simulink model "MEMS_Gyro_Closed_SenseMode_yangchenglunwen"  (R2022b)
settings: Solver=FixedStepAuto  StartTime=0.0  StopTime=5  FixedStep=1/40000  MaxStep=1e-5  RelTol=1e-3
model workspace (MAT data in the model file):
  Ax = 5e-06
  Kamp = 210
  Kcv = 3.5
  Kyc = 114810
  Kyvf = 4.9943e-07
  Qy = 320
  Vr = 2
  Vref = 1
  a0 = 0
  a1 = -1.57079632679
  my = 6.7e-07
  wd = 24001.7678734
  wy = 24416.4581037
  wyx = 24001.7678734
libraries: slpidlib x10, dsparch4 x4
settings Model: Creator=Rio  LastModifiedBy=Rio

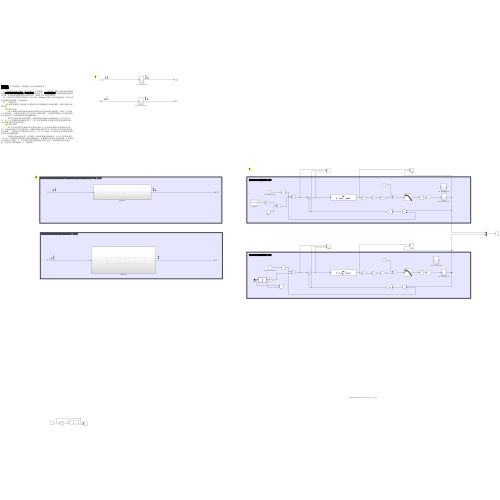
[thumbnail: Simulink's stored preview of the top-level diagram]
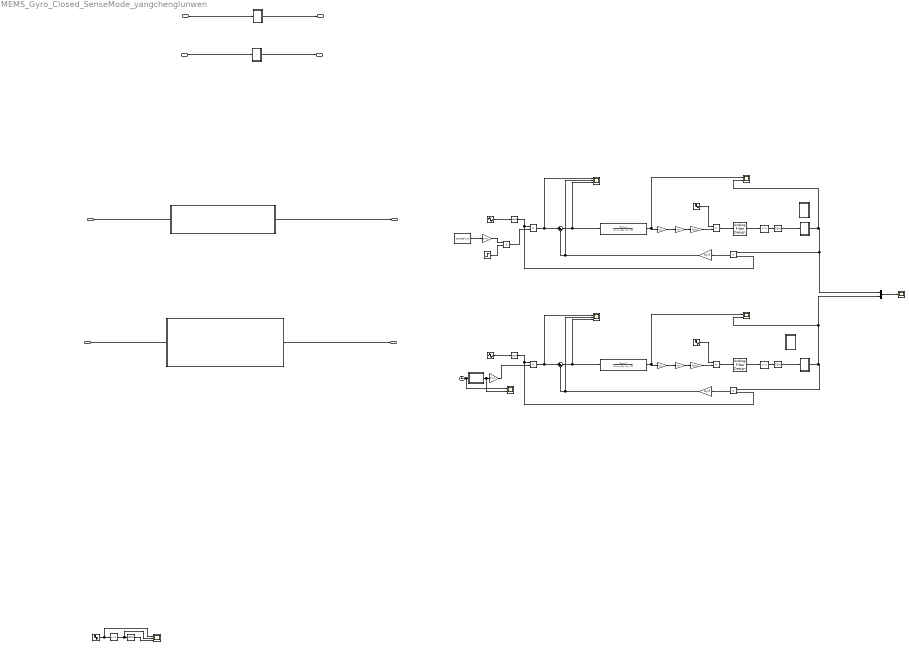
== system MEMS_Gyro_Closed_SenseMode_yangchenglunwen ==
  note: 1
  note: 模态匹配开环检测系统(时域)
  note: 仿真说明 ：参考杨成博士与詹超硕士论文闭环检测仿真
      | 仿真解释 ：
      | 1）闭环检测主要分为两个部分仿真，一个是频域，一个是时域。频域主要看闭环检测系统的 开环传递函数的伯德图、奈奎斯特图 分析稳定性。 闭环的伯德图 可以观察检测系统的带宽性能。时域就是直接观测给定输入信号，观测各个环节的响应情况。
      | 2）当前仿真均在模态匹配状态下进行仿真，即wy=wx,当输入恒定的角速度时，哥氏信号经检测模态相移90°，因此a=-90°。
      | 3）一共3类仿真：
      | 1 中对PI+串联校正器连续以及离散化后的传递函数进行观测伯德图，观察它幅频与相频特性；
      | 2 中有2个仿真：
      | 2.1 从频域传递函数角度观测闭环系统的开环传递函数的伯德图，加校正与不加校正环节的情形（目前仿出来和论文中是对得上的231122）。但是他的零极点与奈奎斯特图与论文相差较远（可能参数哪里有问题231122）。
      | 2.2 同时他的闭环系统伯德图，观测他的输出随输入的幅频特性与论文有很大出入，这一点与时域仿真是相相呼应的。（这与奈奎斯特图以及零极点图的特性是相符合的，因此参数可能还是存在问题）；
      | 3 中有2个仿真：
      | 3.1 首先从时域出发观测在稳定驱动位移信号与恒定角速度输入时系统输出的状态，这时候系统是可以闭环稳定的，检测位移基本被压到了0，加了校正环节后响应速度会有所减慢。（但是矫正环节输出的电压过大，与论文不太相符，可能还是存在参数或者那里结构有些问题231122）
      | 3.2 输入的角速度是有一定的频率，想观测其输出衰减情况，这与论文仿真结果有一定出入。检测反馈力随着输入角速度频率增大，在解调时可能会存在新的问题，这个需要在花些时间去理解一下。这与2.2中闭环的幅频特性是相对应的，说明是哪里还存在着问题，有时间还得仔细琢磨一下（231122）
  note: 观测开环检测输出随输入角速度频率变化，可反应带宽
  note: 3
  note: 模态匹配闭环检测系统的开环传递函数(校正与未校正环节对比)(频域)
  note: 模态匹配闭环检测系统的闭环观测（频域)
  note: 模态匹配开环检测系统(时域)
  note: 2
  Input2 : Inport
  In4 : Inport  Port=2
  Input1 : Inport  Port=3
  In1 : Inport  Port=4
  Analog Filter Design1 : dsparch4/Analog Filter Design  method=Butterworth  filttype=Lowpass  N=2  Wlo=2*pi*150  Whi=80  Rp=2  Rs=40
  Analog Filter Design3 : dsparch4/Analog Filter Design  method=Butterworth  filttype=Lowpass  N=2  Wlo=2*pi*150  Whi=80  Rp=2  Rs=40
  Clock2 : Clock
  Delay1 : Delay  SampleTime=1/1000
  Delay2 : Delay  SampleTime=1/40000
  Delay3 : Delay  SampleTime=1/40000
  Derivative : Derivative
  Derivative4 : Derivative
  Gain : Gain  Gain=2*my
  Gain1 : Gain  Gain=Kcv
  Gain10 : Gain  Gain=Kyc
  Gain11 : Gain  Gain=Kyvf
  Gain2 : Gain  Gain=Kamp
  Gain3 : Gain  Gain=Kyc
  Gain6 : Gain  Gain=Kyvf
  Gain7 : Gain  Gain=2*my
  Gain8 : Gain  Gain=Kcv
  Gain9 : Gain  Gain=Kamp
  MATLAB Function2 : MATLAB Function  TreatAsAtomicUnit=on
  Mux : Mux  Inputs=2
  Product{,1,8..11,13} (7 alike) : Product
  Scope : Scope  NumInputPorts=3
  Scope1 : Scope  NumInputPorts=3
  Scope10 : Scope  NumInputPorts=2
  Scope11 : Scope
  Scope2 : Scope  NumInputPorts=2
  Scope8 : Scope  NumInputPorts=3
  Scope9 : Scope  NumInputPorts=2
  Sine Wave : Sin  Frequency=2*pi*10  SampleTime=0
  Sine Wave1 : Sin  Frequency=wd  SampleTime=1/40000
  Sine Wave5 : Sin  Frequency=wd  SampleTime=1/40000
  Step : Step  SampleTime=1/40000
  Subsystem1 : Subsystem
  Subsystem2 : Subsystem
  Sum : Sum  Inputs=|+-
  Sum1 : Sum  Inputs=|+-
  Transfer Fcn : TransferFcn  Numerator=[1/my]  Denominator=[1 wyx/Qy wyx^2]
  Transfer Fcn2 : TransferFcn  Numerator=[1/my]  Denominator=[1 wyx/Qy wyx^2]
  Zero-Order Hold1 : ZeroOrderHold  SampleTime=1/1000
  Zero-Order Hold2 : ZeroOrderHold  SampleTime=1/40000
  Zero-Order Hold3 : ZeroOrderHold  SampleTime=1/40000
  离散：PI+串联校正器1 : Subsystem
  离散：PI+串联校正器2 : Subsystem
  离散：PI+串联校正器3 : Subsystem
  角速度输入 : Constant  Value=100/360*2*pi  SampleTime=1/40000
  连续：PI+串联校正器1 : Subsystem
  连续：PI+串联校正器2 : Subsystem
  连续：PI+串联校正器3 : Subsystem
  驱动模态速度位移输入 : Sin  Amplitude=Ax  Frequency=wd  SampleTime=1/40000
  驱动模态速度位移输入4 : Sin  Amplitude=Ax  Frequency=wd  SampleTime=1/40000
  Output2 : Outport
  Out4 : Outport  Port=2
  Output1 : Outport  Port=3
  Out1 : Outport  Port=4
  wires:
  Input2/1 -> 连续：PI+串联校正器1/1(u)
  连续：PI+串联校正器1/1(Output2) -> Output2/1
  驱动模态速度位移输入/1 -> Derivative/1
  角速度输入/1 -> Gain/1
  Derivative/1 -> Product9/2, Product/1
  Transfer Fcn/1 -> Gain3/1, Scope2/1
  Gain3/1 -> Gain1/1
  Gain1/1 -> Gain2/1
  Gain2/1 -> Product1/2
  Sine Wave1/1 -> Product1/1
  Product1/1 -> Analog Filter Design3/1
  In4/1 -> Subsystem1/1(In1)
  Subsystem1/1(Output2) -> Out4/1
  离散：PI+串联校正器2/1(Output2) -> Output1/1
  Input1/1 -> 离散：PI+串联校正器2/1(u)
  Delay1/1 -> Scope/2, Zero-Order Hold1/1
  Sine Wave/1 -> Scope/1, Delay1/1
  Zero-Order Hold1/1 -> Scope/3
  Subsystem2/1(Output2) -> Out1/1
  In1/1 -> Subsystem2/1(In1)
  Step/1 -> Product8/2
  Gain/1 -> Product8/1
  Product8/1 -> Product/2
  Product/1 -> Scope1/1, Sum/1
  Sum/1 -> Scope1/3, Transfer Fcn/1
  Product9/1 -> Gain6/1
  Gain6/1 -> Scope1/2, Sum/2
  Delay2/1 -> Zero-Order Hold2/1
  Analog Filter Design3/1 -> Delay2/1
  Zero-Order Hold2/1 -> 离散：PI+串联校正器1/1(u)
  离散：PI+串联校正器1/1(Output2) -> Scope2/2, Mux/1, Product9/1
  离散：PI+串联校正器3/1(Output2) -> Product13/1, Mux/2, Scope9/2
  Zero-Order Hold3/1 -> 离散：PI+串联校正器3/1(u)
  Analog Filter Design1/1 -> Delay3/1
  Delay3/1 -> Zero-Order Hold3/1
  Gain11/1 -> Sum1/2, Scope8/2
  Product13/1 -> Gain11/1
  Sum1/1 -> Transfer Fcn2/1, Scope8/3
  Product10/1 -> Sum1/1, Scope8/1
  Product11/1 -> Analog Filter Design1/1
  Sine Wave5/1 -> Product11/1
  Gain9/1 -> Product11/2
  Gain8/1 -> Gain9/1
  Gain10/1 -> Gain8/1
  Transfer Fcn2/1 -> Scope9/1, Gain10/1
  Derivative4/1 -> Product10/1, Product13/2
  驱动模态速度位移输入4/1 -> Derivative4/1
  MATLAB Function2/1(y) -> Gain7/1, Scope10/2
  Clock2/1 -> MATLAB Function2/1(u), Scope10/1
  Gain7/1 -> Product10/2
  Mux/1 -> Scope11/1

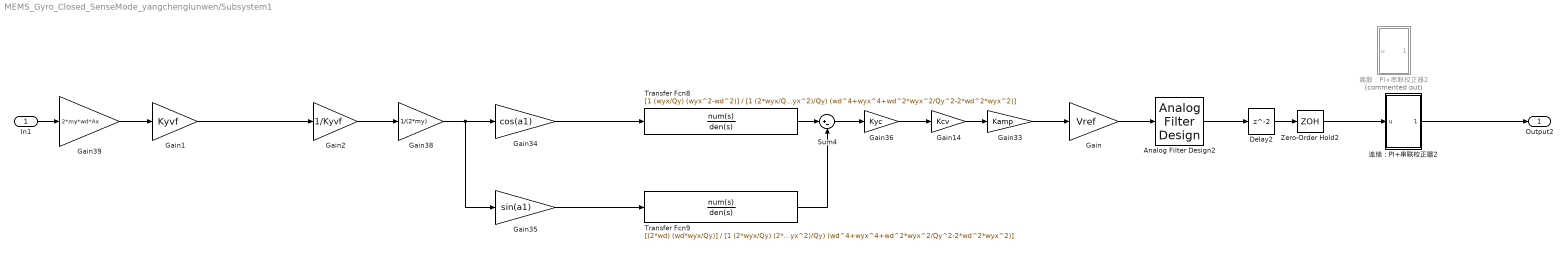
== system MEMS_Gyro_Closed_SenseMode_yangchenglunwen/Subsystem1 ==
  In1 : Inport
  Analog Filter Design2 : dsparch4/Analog Filter Design  method=Butterworth  filttype=Lowpass  N=2  Wlo=2*pi*150  Whi=80  Rp=2  Rs=40
  Delay2 : Delay  SampleTime=1/40000
  Gain : Gain  Gain=Vref
  Gain1 : Gain  Gain=Kyvf
  Gain14 : Gain  Gain=Kcv
  Gain2 : Gain  Gain=1/Kyvf
  Gain33 : Gain  Gain=Kamp
  Gain34 : Gain  Gain=cos(a1)
  Gain35 : Gain  Gain=sin(a1)
  Gain36 : Gain  Gain=Kyc
  Gain38 : Gain  Gain=1/(2*my)
  Gain39 : Gain  Gain=2*my*wd*Ax
  Sum4 : Sum  Inputs=|+-
  Transfer Fcn8 : TransferFcn  Numerator=[1 (wyx/Qy) (wyx^2-wd^2)]  Denominator=[1 (2*wyx/Qy) (2*wd^2+2*wyx^2+wyx^2/Qy^2) (2*wyx*(wd^2+wyx^2)/Qy) (wd^4+wyx^4+wd^2*wyx^2/Qy^2-2*wd^2*wyx^2)]
  Transfer Fcn9 : TransferFcn  Numerator=[(2*wd) (wd*wyx/Qy)]  Denominator=[1 (2*wyx/Qy) (2*wd^2+2*wyx^2+wyx^2/Qy^2) (2*wyx*(wd^2+wyx^2)/Qy) (wd^4+wyx^4+wd^2*wyx^2/Qy^2-2*wd^2*wyx^2)]
  Zero-Order Hold2 : ZeroOrderHold  SampleTime=1/40000
  离散：PI+串联校正器2 : Subsystem  Commented=on
  连续：PI+串联校正器2 : Subsystem
  Output2 : Outport
  wires:
  Analog Filter Design2/1 -> Delay2/1
  Delay2/1 -> Zero-Order Hold2/1
  Sum4/1 -> Gain36/1
  Gain38/1 -> Gain34/1, Gain35/1
  Gain34/1 -> Transfer Fcn8/1
  Transfer Fcn8/1 -> Sum4/1
  Transfer Fcn9/1 -> Sum4/2
  Gain14/1 -> Gain33/1
  Gain35/1 -> Transfer Fcn9/1
  Gain36/1 -> Gain14/1
  In1/1 -> Gain39/1
  Gain33/1 -> Gain/1
  Gain/1 -> Analog Filter Design2/1
  Gain39/1 -> Gain1/1
  Gain2/1 -> Gain38/1
  Zero-Order Hold2/1 -> 连续：PI+串联校正器2/1(u)
  连续：PI+串联校正器2/1(Output2) -> Output2/1
  Gain1/1 -> Gain2/1

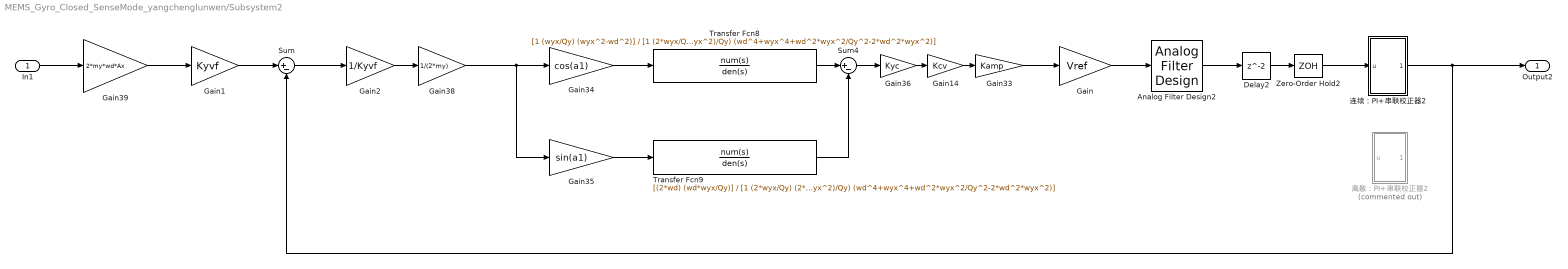
== system MEMS_Gyro_Closed_SenseMode_yangchenglunwen/Subsystem2 ==
  In1 : Inport
  Analog Filter Design2 : dsparch4/Analog Filter Design  method=Butterworth  filttype=Lowpass  N=2  Wlo=2*pi*150  Whi=80  Rp=2  Rs=40
  Delay2 : Delay  SampleTime=1/1000
  Gain : Gain  Gain=Vref
  Gain1 : Gain  Gain=Kyvf
  Gain14 : Gain  Gain=Kcv
  Gain2 : Gain  Gain=1/Kyvf
  Gain33 : Gain  Gain=Kamp
  Gain34 : Gain  Gain=cos(a1)
  Gain35 : Gain  Gain=sin(a1)
  Gain36 : Gain  Gain=Kyc
  Gain38 : Gain  Gain=1/(2*my)
  Gain39 : Gain  Gain=2*my*wd*Ax
  Sum : Sum  Inputs=|+-
  Sum4 : Sum  Inputs=|+-
  Transfer Fcn8 : TransferFcn  Numerator=[1 (wyx/Qy) (wyx^2-wd^2)]  Denominator=[1 (2*wyx/Qy) (2*wd^2+2*wyx^2+wyx^2/Qy^2) (2*wyx*(wd^2+wyx^2)/Qy) (wd^4+wyx^4+wd^2*wyx^2/Qy^2-2*wd^2*wyx^2)]
  Transfer Fcn9 : TransferFcn  Numerator=[(2*wd) (wd*wyx/Qy)]  Denominator=[1 (2*wyx/Qy) (2*wd^2+2*wyx^2+wyx^2/Qy^2) (2*wyx*(wd^2+wyx^2)/Qy) (wd^4+wyx^4+wd^2*wyx^2/Qy^2-2*wd^2*wyx^2)]
  Zero-Order Hold2 : ZeroOrderHold  SampleTime=1/1000
  离散：PI+串联校正器2 : Subsystem  Commented=on
  连续：PI+串联校正器2 : Subsystem
  Output2 : Outport
  wires:
  Analog Filter Design2/1 -> Delay2/1
  Gain/1 -> Analog Filter Design2/1
  Gain33/1 -> Gain/1
  In1/1 -> Gain39/1
  Sum4/1 -> Gain36/1
  Gain36/1 -> Gain14/1
  Gain34/1 -> Transfer Fcn8/1
  Gain35/1 -> Transfer Fcn9/1
  Transfer Fcn9/1 -> Sum4/2
  Transfer Fcn8/1 -> Sum4/1
  Delay2/1 -> Zero-Order Hold2/1
  连续：PI+串联校正器2/1(Output2) -> Sum/2, Output2/1
  Gain14/1 -> Gain33/1
  Gain38/1 -> Gain35/1, Gain34/1
  Zero-Order Hold2/1 -> 连续：PI+串联校正器2/1(u)
  Gain39/1 -> Gain1/1
  Gain1/1 -> Sum/1
  Gain2/1 -> Gain38/1
  Sum/1 -> Gain2/1

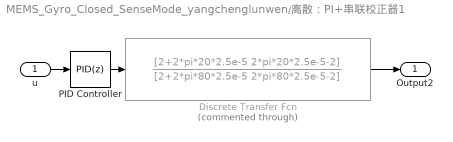
== system MEMS_Gyro_Closed_SenseMode_yangchenglunwen/离散：PI+串联校正器1 ==
  u : Inport
  Discrete Transfer Fcn : DiscreteTransferFcn  Commented=through  Numerator=[2+2*pi*20*2.5e-5 2*pi*20*2.5e-5-2]  Denominator=[2+2*pi*80*2.5e-5 2*pi*80*2.5e-5-2]  SampleTime=1/40000
  PID Controller : slpidlib/PID Controller  Controller=PID  Form=Parallel  TimeDomain=Discrete-time  UseExternalTs=off  SampleTime=1/40000  IntegratorMethod=Forward Euler  FilterMethod=Forward Euler  ControllerParametersSource=internal  P=0.1  I=2*pi*20  UseKiTs=off  D=0  N=100  UseFilter=on  TunerSelectOption=Transfer Function Based (PID Tuner App)  InitialConditionSource=internal  InitialConditionForIntegrator=0  InitialConditionForFilter=0  DifferentiatorICPrevScaledInput=0  ExternalReset=none  TrackingMode=off  Kt=1  LimitOutput=off  SatLimitsSource=internal  UpperSaturationLimit=inf  LowerSaturationLimit=-inf  LinearizeAsGain=on  AntiWindupMode=none  Kb=1  LimitIntegrator=off  UpperIntegratorSaturationLimit=inf  LowerIntegratorSaturationLimit=-inf  POutMin=[]  POutMax=[]  IOutMin=[]  IOutMax=[]  DOutMin=[]  DOutMax=[]  NOutMin=[]  NOutMax=[]  SumOutMin=[]  SumOutMax=[]  SaturationOutMin=[]  SaturationOutMax=[]  PParamMin=[]  PParamMax=[]  IParamMin=[]  IParamMax=[]  DParamMin=[]  DParamMax=[]  NParamMin=[]  NParamMax=[]  KbParamMin=[]  KbParamMax=[]  KtParamMin=[]  KtParamMax=[]  KbOutMin=[]  KbOutMax=[]  KtOutMin=[]  KtOutMax=[]  IntegratorOutMin=[]  IntegratorOutMax=[]  FilterOutMin=[]  FilterOutMax=[]  SumI1OutMin=[]  SumI1OutMax=[]  SumI2OutMin=[]  SumI2OutMax=[]  SumI3OutMin=[]  SumI3OutMax=[]  SumI4OutMin=[]  SumI4OutMax=[]  SumDOutMin=[]  SumDOutMax=[]  DifferentiatorOutMin=[]  DifferentiatorOutMax=[]  FilterDiffOutCoefMin=[]  FilterDiffOutCoefMax=[]  ReciprocalOutMin=[]  ReciprocalOutMax=[]  SumDenOutMin=[]  SumDenOutMax=[]  SumNumOutMin=[]  SumNumOutMax=[]  DivideOutMin=[]  DivideOutMax=[]  UdiffTsProdOutMin=[]  UdiffTsProdOutMax=[]  NTsProdOutMin=[]  NTsProdOutMax=[]  UintegralTsProdOutMin=[]  UintegralTsProdOutMax=[]  UngainTsProdOutMin=[]  UngainTsProdOutMax=[]  ClampingZeroOutDataTypeStr=Inherit: Inherit via back propagation  ClampingZeroOutMin=[]  ClampingZeroOutMax=[]  FilterDenConstantOutDataTypeStr=Inherit: Inherit via back propagation  FilterDenConstantOutMin=[]  FilterDenConstantOutMax=[]  PCopyOutDataTypeStr=Inherit: Inherit via back propagation  PCopyOutMin=[]  PCopyOutMax=[]  NCopyOutDataTypeStr=Inherit: Inherit via back propagation  NCopyOutMin=[]  NCopyOutMax=[]  IntegratorContinuousStateAttributes=''  IntegratorStateMustResolveToSignalObject=off  IntegratorRTWStateStorageClass=Auto  FilterContinuousStateAttributes=''  FilterStateMustResolveToSignalObject=off  FilterRTWStateStorageClass=Auto  ParallelPVariant=InternalParameters  IdealPVariant=Disabled  IVariant=InternalParameters  DVariant=InternalParameters  IntegratorVariant=Discrete  SatVariant=Disabled  AWVariant=Passthrough  PCopyVariant=Disabled  TRVariant=Disabled  FdbkBlocksVariant=Forward  IdealPFdbkVariant=Disabled  SatFdbkVariant=Disabled  DerivativeFilterVariant=ForwardEulerFilter  NVariant=InternalParameters  NCopyVariant=Disabled  FilterICVariant=InternalICsFilter  IntegratorICVariant=InternalICs  ExternalResetVariant=Disabled  TRSumVariant=Passthrough  SumFdbkVariant=Disabled  SumVariant=Sum_PID  TsampFilterVariant=InternalTs  TsampNgainVariant=Passthrough  TsampIntegralVariant=Passthrough  ExternalSaturationOutDataTypeStr=Inherit: Same as second input
  Output2 : Outport
  wires:
  Discrete Transfer Fcn/1 -> Output2/1
  PID Controller/1 -> Discrete Transfer Fcn/1
  u/1 -> PID Controller/1

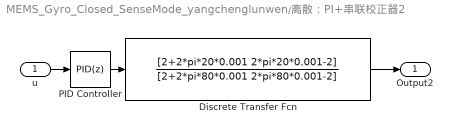
== system MEMS_Gyro_Closed_SenseMode_yangchenglunwen/离散：PI+串联校正器2 ==
  u : Inport
  Discrete Transfer Fcn : DiscreteTransferFcn  Numerator=[2+2*pi*20*0.001 2*pi*20*0.001-2]  Denominator=[2+2*pi*80*0.001 2*pi*80*0.001-2]
  PID Controller : slpidlib/PID Controller  Controller=PID  Form=Parallel  TimeDomain=Discrete-time  UseExternalTs=off  SampleTime=1/1000  IntegratorMethod=Forward Euler  FilterMethod=Forward Euler  ControllerParametersSource=internal  P=0.9  I=2*pi*18  UseKiTs=off  D=0  N=100  UseFilter=on  TunerSelectOption=Transfer Function Based (PID Tuner App)  InitialConditionSource=internal  InitialConditionForIntegrator=0  InitialConditionForFilter=0  DifferentiatorICPrevScaledInput=0  ExternalReset=none  TrackingMode=off  Kt=1  LimitOutput=off  SatLimitsSource=internal  UpperSaturationLimit=inf  LowerSaturationLimit=-inf  LinearizeAsGain=on  AntiWindupMode=none  Kb=1  LimitIntegrator=off  UpperIntegratorSaturationLimit=inf  LowerIntegratorSaturationLimit=-inf  POutMin=[]  POutMax=[]  IOutMin=[]  IOutMax=[]  DOutMin=[]  DOutMax=[]  NOutMin=[]  NOutMax=[]  SumOutMin=[]  SumOutMax=[]  SaturationOutMin=[]  SaturationOutMax=[]  PParamMin=[]  PParamMax=[]  IParamMin=[]  IParamMax=[]  DParamMin=[]  DParamMax=[]  NParamMin=[]  NParamMax=[]  KbParamMin=[]  KbParamMax=[]  KtParamMin=[]  KtParamMax=[]  KbOutMin=[]  KbOutMax=[]  KtOutMin=[]  KtOutMax=[]  IntegratorOutMin=[]  IntegratorOutMax=[]  FilterOutMin=[]  FilterOutMax=[]  SumI1OutMin=[]  SumI1OutMax=[]  SumI2OutMin=[]  SumI2OutMax=[]  SumI3OutMin=[]  SumI3OutMax=[]  SumI4OutMin=[]  SumI4OutMax=[]  SumDOutMin=[]  SumDOutMax=[]  DifferentiatorOutMin=[]  DifferentiatorOutMax=[]  FilterDiffOutCoefMin=[]  FilterDiffOutCoefMax=[]  ReciprocalOutMin=[]  ReciprocalOutMax=[]  SumDenOutMin=[]  SumDenOutMax=[]  SumNumOutMin=[]  SumNumOutMax=[]  DivideOutMin=[]  DivideOutMax=[]  UdiffTsProdOutMin=[]  UdiffTsProdOutMax=[]  NTsProdOutMin=[]  NTsProdOutMax=[]  UintegralTsProdOutMin=[]  UintegralTsProdOutMax=[]  UngainTsProdOutMin=[]  UngainTsProdOutMax=[]  ClampingZeroOutDataTypeStr=Inherit: Inherit via back propagation  ClampingZeroOutMin=[]  ClampingZeroOutMax=[]  FilterDenConstantOutDataTypeStr=Inherit: Inherit via back propagation  FilterDenConstantOutMin=[]  FilterDenConstantOutMax=[]  PCopyOutDataTypeStr=Inherit: Inherit via back propagation  PCopyOutMin=[]  PCopyOutMax=[]  NCopyOutDataTypeStr=Inherit: Inherit via back propagation  NCopyOutMin=[]  NCopyOutMax=[]  IntegratorContinuousStateAttributes=''  IntegratorStateMustResolveToSignalObject=off  IntegratorRTWStateStorageClass=Auto  FilterContinuousStateAttributes=''  FilterStateMustResolveToSignalObject=off  FilterRTWStateStorageClass=Auto  ParallelPVariant=InternalParameters  IdealPVariant=Disabled  IVariant=InternalParameters  DVariant=InternalParameters  IntegratorVariant=Discrete  SatVariant=Disabled  AWVariant=Passthrough  PCopyVariant=Disabled  TRVariant=Disabled  FdbkBlocksVariant=Forward  IdealPFdbkVariant=Disabled  SatFdbkVariant=Disabled  DerivativeFilterVariant=ForwardEulerFilter  NVariant=InternalParameters  NCopyVariant=Disabled  FilterICVariant=InternalICsFilter  IntegratorICVariant=InternalICs  ExternalResetVariant=Disabled  TRSumVariant=Passthrough  SumFdbkVariant=Disabled  SumVariant=Sum_PID  TsampFilterVariant=InternalTs  TsampNgainVariant=Passthrough  TsampIntegralVariant=Passthrough  ExternalSaturationOutDataTypeStr=Inherit: Same as second input
  Output2 : Outport
  wires:
  u/1 -> PID Controller/1
  PID Controller/1 -> Discrete Transfer Fcn/1
  Discrete Transfer Fcn/1 -> Output2/1

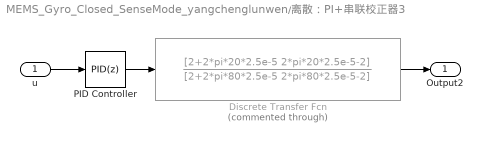
== system MEMS_Gyro_Closed_SenseMode_yangchenglunwen/离散：PI+串联校正器3 ==
  u : Inport
  Discrete Transfer Fcn : DiscreteTransferFcn  Commented=through  Numerator=[2+2*pi*20*2.5e-5 2*pi*20*2.5e-5-2]  Denominator=[2+2*pi*80*2.5e-5 2*pi*80*2.5e-5-2]  SampleTime=1/40000
  PID Controller : slpidlib/PID Controller  Controller=PID  Form=Parallel  TimeDomain=Discrete-time  UseExternalTs=off  SampleTime=1/40000  IntegratorMethod=Forward Euler  FilterMethod=Forward Euler  ControllerParametersSource=internal  P=0.1  I=2*pi*20  UseKiTs=off  D=0  N=100  UseFilter=on  TunerSelectOption=Transfer Function Based (PID Tuner App)  InitialConditionSource=internal  InitialConditionForIntegrator=0  InitialConditionForFilter=0  DifferentiatorICPrevScaledInput=0  ExternalReset=none  TrackingMode=off  Kt=1  LimitOutput=off  SatLimitsSource=internal  UpperSaturationLimit=inf  LowerSaturationLimit=-inf  LinearizeAsGain=on  AntiWindupMode=none  Kb=1  LimitIntegrator=off  UpperIntegratorSaturationLimit=inf  LowerIntegratorSaturationLimit=-inf  POutMin=[]  POutMax=[]  IOutMin=[]  IOutMax=[]  DOutMin=[]  DOutMax=[]  NOutMin=[]  NOutMax=[]  SumOutMin=[]  SumOutMax=[]  SaturationOutMin=[]  SaturationOutMax=[]  PParamMin=[]  PParamMax=[]  IParamMin=[]  IParamMax=[]  DParamMin=[]  DParamMax=[]  NParamMin=[]  NParamMax=[]  KbParamMin=[]  KbParamMax=[]  KtParamMin=[]  KtParamMax=[]  KbOutMin=[]  KbOutMax=[]  KtOutMin=[]  KtOutMax=[]  IntegratorOutMin=[]  IntegratorOutMax=[]  FilterOutMin=[]  FilterOutMax=[]  SumI1OutMin=[]  SumI1OutMax=[]  SumI2OutMin=[]  SumI2OutMax=[]  SumI3OutMin=[]  SumI3OutMax=[]  SumI4OutMin=[]  SumI4OutMax=[]  SumDOutMin=[]  SumDOutMax=[]  DifferentiatorOutMin=[]  DifferentiatorOutMax=[]  FilterDiffOutCoefMin=[]  FilterDiffOutCoefMax=[]  ReciprocalOutMin=[]  ReciprocalOutMax=[]  SumDenOutMin=[]  SumDenOutMax=[]  SumNumOutMin=[]  SumNumOutMax=[]  DivideOutMin=[]  DivideOutMax=[]  UdiffTsProdOutMin=[]  UdiffTsProdOutMax=[]  NTsProdOutMin=[]  NTsProdOutMax=[]  UintegralTsProdOutMin=[]  UintegralTsProdOutMax=[]  UngainTsProdOutMin=[]  UngainTsProdOutMax=[]  ClampingZeroOutDataTypeStr=Inherit: Inherit via back propagation  ClampingZeroOutMin=[]  ClampingZeroOutMax=[]  FilterDenConstantOutDataTypeStr=Inherit: Inherit via back propagation  FilterDenConstantOutMin=[]  FilterDenConstantOutMax=[]  PCopyOutDataTypeStr=Inherit: Inherit via back propagation  PCopyOutMin=[]  PCopyOutMax=[]  NCopyOutDataTypeStr=Inherit: Inherit via back propagation  NCopyOutMin=[]  NCopyOutMax=[]  IntegratorContinuousStateAttributes=''  IntegratorStateMustResolveToSignalObject=off  IntegratorRTWStateStorageClass=Auto  FilterContinuousStateAttributes=''  FilterStateMustResolveToSignalObject=off  FilterRTWStateStorageClass=Auto  ParallelPVariant=InternalParameters  IdealPVariant=Disabled  IVariant=InternalParameters  DVariant=InternalParameters  IntegratorVariant=Discrete  SatVariant=Disabled  AWVariant=Passthrough  PCopyVariant=Disabled  TRVariant=Disabled  FdbkBlocksVariant=Forward  IdealPFdbkVariant=Disabled  SatFdbkVariant=Disabled  DerivativeFilterVariant=ForwardEulerFilter  NVariant=InternalParameters  NCopyVariant=Disabled  FilterICVariant=InternalICsFilter  IntegratorICVariant=InternalICs  ExternalResetVariant=Disabled  TRSumVariant=Passthrough  SumFdbkVariant=Disabled  SumVariant=Sum_PID  TsampFilterVariant=InternalTs  TsampNgainVariant=Passthrough  TsampIntegralVariant=Passthrough  ExternalSaturationOutDataTypeStr=Inherit: Same as second input
  Output2 : Outport
  wires:
  u/1 -> PID Controller/1
  PID Controller/1 -> Discrete Transfer Fcn/1
  Discrete Transfer Fcn/1 -> Output2/1

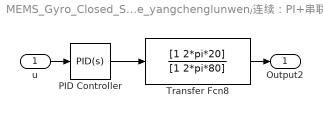
== system MEMS_Gyro_Closed_SenseMode_yangchenglunwen/连续：PI+串联校正器1 ==
  u : Inport
  PID Controller : slpidlib/PID Controller  Controller=PID  Form=Parallel  TimeDomain=Continuous-time  UseExternalTs=off  SampleTime=-1  IntegratorMethod=Forward Euler  FilterMethod=Forward Euler  ControllerParametersSource=internal  P=0.9  I=2*pi*18  UseKiTs=off  D=0  N=100  UseFilter=on  TunerSelectOption=Transfer Function Based (PID Tuner App)  InitialConditionSource=internal  InitialConditionForIntegrator=0  InitialConditionForFilter=0  DifferentiatorICPrevScaledInput=0  ExternalReset=none  TrackingMode=off  Kt=1  LimitOutput=off  SatLimitsSource=internal  UpperSaturationLimit=inf  LowerSaturationLimit=-inf  LinearizeAsGain=on  AntiWindupMode=none  Kb=1  LimitIntegrator=off  UpperIntegratorSaturationLimit=inf  LowerIntegratorSaturationLimit=-inf  POutMin=[]  POutMax=[]  IOutMin=[]  IOutMax=[]  DOutMin=[]  DOutMax=[]  NOutMin=[]  NOutMax=[]  SumOutMin=[]  SumOutMax=[]  SaturationOutMin=[]  SaturationOutMax=[]  PParamMin=[]  PParamMax=[]  IParamMin=[]  IParamMax=[]  DParamMin=[]  DParamMax=[]  NParamMin=[]  NParamMax=[]  KbParamMin=[]  KbParamMax=[]  KtParamMin=[]  KtParamMax=[]  KbOutMin=[]  KbOutMax=[]  KtOutMin=[]  KtOutMax=[]  IntegratorOutMin=[]  IntegratorOutMax=[]  FilterOutMin=[]  FilterOutMax=[]  SumI1OutMin=[]  SumI1OutMax=[]  SumI2OutMin=[]  SumI2OutMax=[]  SumI3OutMin=[]  SumI3OutMax=[]  SumI4OutMin=[]  SumI4OutMax=[]  SumDOutMin=[]  SumDOutMax=[]  DifferentiatorOutMin=[]  DifferentiatorOutMax=[]  FilterDiffOutCoefMin=[]  FilterDiffOutCoefMax=[]  ReciprocalOutMin=[]  ReciprocalOutMax=[]  SumDenOutMin=[]  SumDenOutMax=[]  SumNumOutMin=[]  SumNumOutMax=[]  DivideOutMin=[]  DivideOutMax=[]  UdiffTsProdOutMin=[]  UdiffTsProdOutMax=[]  NTsProdOutMin=[]  NTsProdOutMax=[]  UintegralTsProdOutMin=[]  UintegralTsProdOutMax=[]  UngainTsProdOutMin=[]  UngainTsProdOutMax=[]  ClampingZeroOutDataTypeStr=Inherit: Inherit via back propagation  ClampingZeroOutMin=[]  ClampingZeroOutMax=[]  FilterDenConstantOutDataTypeStr=Inherit: Inherit via back propagation  FilterDenConstantOutMin=[]  FilterDenConstantOutMax=[]  PCopyOutDataTypeStr=Inherit: Inherit via back propagation  PCopyOutMin=[]  PCopyOutMax=[]  NCopyOutDataTypeStr=Inherit: Inherit via back propagation  NCopyOutMin=[]  NCopyOutMax=[]  IntegratorContinuousStateAttributes=''  IntegratorStateMustResolveToSignalObject=off  IntegratorRTWStateStorageClass=Auto  FilterContinuousStateAttributes=''  FilterStateMustResolveToSignalObject=off  FilterRTWStateStorageClass=Auto  ParallelPVariant=InternalParameters  IdealPVariant=Disabled  IVariant=InternalParameters  DVariant=InternalParameters  IntegratorVariant=Continuous  SatVariant=Disabled  AWVariant=Passthrough  PCopyVariant=Disabled  TRVariant=Disabled  FdbkBlocksVariant=Forward  IdealPFdbkVariant=Disabled  SatFdbkVariant=Disabled  DerivativeFilterVariant=ContFilter  NVariant=InternalParameters  NCopyVariant=Disabled  FilterICVariant=InternalICsFilter  IntegratorICVariant=InternalICs  ExternalResetVariant=Disabled  TRSumVariant=Passthrough  SumFdbkVariant=Disabled  SumVariant=Sum_PID  TsampFilterVariant=InternalTs  TsampNgainVariant=Passthrough  TsampIntegralVariant=Passthrough  ExternalSaturationOutDataTypeStr=Inherit: Same as second input
  Transfer Fcn8 : TransferFcn  Numerator=[1 2*pi*20]  Denominator=[1 2*pi*80]
  Output2 : Outport
  wires:
  Transfer Fcn8/1 -> Output2/1
  PID Controller/1 -> Transfer Fcn8/1
  u/1 -> PID Controller/1

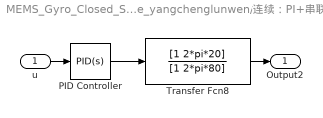
== system MEMS_Gyro_Closed_SenseMode_yangchenglunwen/连续：PI+串联校正器2 ==
  u : Inport
  PID Controller : slpidlib/PID Controller  Controller=PID  Form=Parallel  TimeDomain=Continuous-time  UseExternalTs=off  SampleTime=-1  IntegratorMethod=Forward Euler  FilterMethod=Forward Euler  ControllerParametersSource=internal  P=0.9  I=2*pi*18  UseKiTs=off  D=0  N=100  UseFilter=on  TunerSelectOption=Transfer Function Based (PID Tuner App)  InitialConditionSource=internal  InitialConditionForIntegrator=0  InitialConditionForFilter=0  DifferentiatorICPrevScaledInput=0  ExternalReset=none  TrackingMode=off  Kt=1  LimitOutput=off  SatLimitsSource=internal  UpperSaturationLimit=inf  LowerSaturationLimit=-inf  LinearizeAsGain=on  AntiWindupMode=none  Kb=1  LimitIntegrator=off  UpperIntegratorSaturationLimit=inf  LowerIntegratorSaturationLimit=-inf  POutMin=[]  POutMax=[]  IOutMin=[]  IOutMax=[]  DOutMin=[]  DOutMax=[]  NOutMin=[]  NOutMax=[]  SumOutMin=[]  SumOutMax=[]  SaturationOutMin=[]  SaturationOutMax=[]  PParamMin=[]  PParamMax=[]  IParamMin=[]  IParamMax=[]  DParamMin=[]  DParamMax=[]  NParamMin=[]  NParamMax=[]  KbParamMin=[]  KbParamMax=[]  KtParamMin=[]  KtParamMax=[]  KbOutMin=[]  KbOutMax=[]  KtOutMin=[]  KtOutMax=[]  IntegratorOutMin=[]  IntegratorOutMax=[]  FilterOutMin=[]  FilterOutMax=[]  SumI1OutMin=[]  SumI1OutMax=[]  SumI2OutMin=[]  SumI2OutMax=[]  SumI3OutMin=[]  SumI3OutMax=[]  SumI4OutMin=[]  SumI4OutMax=[]  SumDOutMin=[]  SumDOutMax=[]  DifferentiatorOutMin=[]  DifferentiatorOutMax=[]  FilterDiffOutCoefMin=[]  FilterDiffOutCoefMax=[]  ReciprocalOutMin=[]  ReciprocalOutMax=[]  SumDenOutMin=[]  SumDenOutMax=[]  SumNumOutMin=[]  SumNumOutMax=[]  DivideOutMin=[]  DivideOutMax=[]  UdiffTsProdOutMin=[]  UdiffTsProdOutMax=[]  NTsProdOutMin=[]  NTsProdOutMax=[]  UintegralTsProdOutMin=[]  UintegralTsProdOutMax=[]  UngainTsProdOutMin=[]  UngainTsProdOutMax=[]  ClampingZeroOutDataTypeStr=Inherit: Inherit via back propagation  ClampingZeroOutMin=[]  ClampingZeroOutMax=[]  FilterDenConstantOutDataTypeStr=Inherit: Inherit via back propagation  FilterDenConstantOutMin=[]  FilterDenConstantOutMax=[]  PCopyOutDataTypeStr=Inherit: Inherit via back propagation  PCopyOutMin=[]  PCopyOutMax=[]  NCopyOutDataTypeStr=Inherit: Inherit via back propagation  NCopyOutMin=[]  NCopyOutMax=[]  IntegratorContinuousStateAttributes=''  IntegratorStateMustResolveToSignalObject=off  IntegratorRTWStateStorageClass=Auto  FilterContinuousStateAttributes=''  FilterStateMustResolveToSignalObject=off  FilterRTWStateStorageClass=Auto  ParallelPVariant=InternalParameters  IdealPVariant=Disabled  IVariant=InternalParameters  DVariant=InternalParameters  IntegratorVariant=Continuous  SatVariant=Disabled  AWVariant=Passthrough  PCopyVariant=Disabled  TRVariant=Disabled  FdbkBlocksVariant=Forward  IdealPFdbkVariant=Disabled  SatFdbkVariant=Disabled  DerivativeFilterVariant=ContFilter  NVariant=InternalParameters  NCopyVariant=Disabled  FilterICVariant=InternalICsFilter  IntegratorICVariant=InternalICs  ExternalResetVariant=Disabled  TRSumVariant=Passthrough  SumFdbkVariant=Disabled  SumVariant=Sum_PID  TsampFilterVariant=InternalTs  TsampNgainVariant=Passthrough  TsampIntegralVariant=Passthrough  ExternalSaturationOutDataTypeStr=Inherit: Same as second input
  Transfer Fcn8 : TransferFcn  Numerator=[1 2*pi*20]  Denominator=[1 2*pi*80]
  Output2 : Outport
  wires:
  u/1 -> PID Controller/1
  PID Controller/1 -> Transfer Fcn8/1
  Transfer Fcn8/1 -> Output2/1

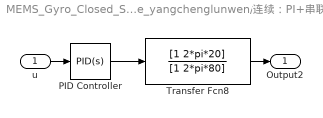
== system MEMS_Gyro_Closed_SenseMode_yangchenglunwen/连续：PI+串联校正器3 ==
  u : Inport
  PID Controller : slpidlib/PID Controller  Controller=PID  Form=Parallel  TimeDomain=Continuous-time  UseExternalTs=off  SampleTime=-1  IntegratorMethod=Forward Euler  FilterMethod=Forward Euler  ControllerParametersSource=internal  P=0.9  I=2*pi*18  UseKiTs=off  D=0  N=100  UseFilter=on  TunerSelectOption=Transfer Function Based (PID Tuner App)  InitialConditionSource=internal  InitialConditionForIntegrator=0  InitialConditionForFilter=0  DifferentiatorICPrevScaledInput=0  ExternalReset=none  TrackingMode=off  Kt=1  LimitOutput=off  SatLimitsSource=internal  UpperSaturationLimit=inf  LowerSaturationLimit=-inf  LinearizeAsGain=on  AntiWindupMode=none  Kb=1  LimitIntegrator=off  UpperIntegratorSaturationLimit=inf  LowerIntegratorSaturationLimit=-inf  POutMin=[]  POutMax=[]  IOutMin=[]  IOutMax=[]  DOutMin=[]  DOutMax=[]  NOutMin=[]  NOutMax=[]  SumOutMin=[]  SumOutMax=[]  SaturationOutMin=[]  SaturationOutMax=[]  PParamMin=[]  PParamMax=[]  IParamMin=[]  IParamMax=[]  DParamMin=[]  DParamMax=[]  NParamMin=[]  NParamMax=[]  KbParamMin=[]  KbParamMax=[]  KtParamMin=[]  KtParamMax=[]  KbOutMin=[]  KbOutMax=[]  KtOutMin=[]  KtOutMax=[]  IntegratorOutMin=[]  IntegratorOutMax=[]  FilterOutMin=[]  FilterOutMax=[]  SumI1OutMin=[]  SumI1OutMax=[]  SumI2OutMin=[]  SumI2OutMax=[]  SumI3OutMin=[]  SumI3OutMax=[]  SumI4OutMin=[]  SumI4OutMax=[]  SumDOutMin=[]  SumDOutMax=[]  DifferentiatorOutMin=[]  DifferentiatorOutMax=[]  FilterDiffOutCoefMin=[]  FilterDiffOutCoefMax=[]  ReciprocalOutMin=[]  ReciprocalOutMax=[]  SumDenOutMin=[]  SumDenOutMax=[]  SumNumOutMin=[]  SumNumOutMax=[]  DivideOutMin=[]  DivideOutMax=[]  UdiffTsProdOutMin=[]  UdiffTsProdOutMax=[]  NTsProdOutMin=[]  NTsProdOutMax=[]  UintegralTsProdOutMin=[]  UintegralTsProdOutMax=[]  UngainTsProdOutMin=[]  UngainTsProdOutMax=[]  ClampingZeroOutDataTypeStr=Inherit: Inherit via back propagation  ClampingZeroOutMin=[]  ClampingZeroOutMax=[]  FilterDenConstantOutDataTypeStr=Inherit: Inherit via back propagation  FilterDenConstantOutMin=[]  FilterDenConstantOutMax=[]  PCopyOutDataTypeStr=Inherit: Inherit via back propagation  PCopyOutMin=[]  PCopyOutMax=[]  NCopyOutDataTypeStr=Inherit: Inherit via back propagation  NCopyOutMin=[]  NCopyOutMax=[]  IntegratorContinuousStateAttributes=''  IntegratorStateMustResolveToSignalObject=off  IntegratorRTWStateStorageClass=Auto  FilterContinuousStateAttributes=''  FilterStateMustResolveToSignalObject=off  FilterRTWStateStorageClass=Auto  ParallelPVariant=InternalParameters  IdealPVariant=Disabled  IVariant=InternalParameters  DVariant=InternalParameters  IntegratorVariant=Continuous  SatVariant=Disabled  AWVariant=Passthrough  PCopyVariant=Disabled  TRVariant=Disabled  FdbkBlocksVariant=Forward  IdealPFdbkVariant=Disabled  SatFdbkVariant=Disabled  DerivativeFilterVariant=ContFilter  NVariant=InternalParameters  NCopyVariant=Disabled  FilterICVariant=InternalICsFilter  IntegratorICVariant=InternalICs  ExternalResetVariant=Disabled  TRSumVariant=Passthrough  SumFdbkVariant=Disabled  SumVariant=Sum_PID  TsampFilterVariant=InternalTs  TsampNgainVariant=Passthrough  TsampIntegralVariant=Passthrough  ExternalSaturationOutDataTypeStr=Inherit: Same as second input
  Transfer Fcn8 : TransferFcn  Numerator=[1 2*pi*20]  Denominator=[1 2*pi*80]
  Output2 : Outport
  wires:
  Transfer Fcn8/1 -> Output2/1
  PID Controller/1 -> Transfer Fcn8/1
  u/1 -> PID Controller/1

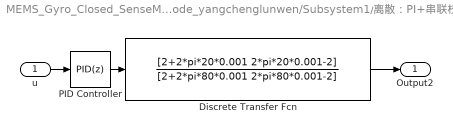
== system MEMS_Gyro_Closed_SenseMode_yangchenglunwen/Subsystem1/离散：PI+串联校正器2 ==
  u : Inport
  Discrete Transfer Fcn : DiscreteTransferFcn  Numerator=[2+2*pi*20*0.001 2*pi*20*0.001-2]  Denominator=[2+2*pi*80*0.001 2*pi*80*0.001-2]  SampleTime=1/1000
  PID Controller : slpidlib/PID Controller  Controller=PID  Form=Parallel  TimeDomain=Discrete-time  UseExternalTs=off  SampleTime=1/1000  IntegratorMethod=Forward Euler  FilterMethod=Forward Euler  ControllerParametersSource=internal  P=0.9  I=2*pi*18  UseKiTs=off  D=0  N=100  UseFilter=on  TunerSelectOption=Transfer Function Based (PID Tuner App)  InitialConditionSource=internal  InitialConditionForIntegrator=0  InitialConditionForFilter=0  DifferentiatorICPrevScaledInput=0  ExternalReset=none  TrackingMode=off  Kt=1  LimitOutput=off  SatLimitsSource=internal  UpperSaturationLimit=inf  LowerSaturationLimit=-inf  LinearizeAsGain=on  AntiWindupMode=none  Kb=1  LimitIntegrator=off  UpperIntegratorSaturationLimit=inf  LowerIntegratorSaturationLimit=-inf  POutMin=[]  POutMax=[]  IOutMin=[]  IOutMax=[]  DOutMin=[]  DOutMax=[]  NOutMin=[]  NOutMax=[]  SumOutMin=[]  SumOutMax=[]  SaturationOutMin=[]  SaturationOutMax=[]  PParamMin=[]  PParamMax=[]  IParamMin=[]  IParamMax=[]  DParamMin=[]  DParamMax=[]  NParamMin=[]  NParamMax=[]  KbParamMin=[]  KbParamMax=[]  KtParamMin=[]  KtParamMax=[]  KbOutMin=[]  KbOutMax=[]  KtOutMin=[]  KtOutMax=[]  IntegratorOutMin=[]  IntegratorOutMax=[]  FilterOutMin=[]  FilterOutMax=[]  SumI1OutMin=[]  SumI1OutMax=[]  SumI2OutMin=[]  SumI2OutMax=[]  SumI3OutMin=[]  SumI3OutMax=[]  SumI4OutMin=[]  SumI4OutMax=[]  SumDOutMin=[]  SumDOutMax=[]  DifferentiatorOutMin=[]  DifferentiatorOutMax=[]  FilterDiffOutCoefMin=[]  FilterDiffOutCoefMax=[]  ReciprocalOutMin=[]  ReciprocalOutMax=[]  SumDenOutMin=[]  SumDenOutMax=[]  SumNumOutMin=[]  SumNumOutMax=[]  DivideOutMin=[]  DivideOutMax=[]  UdiffTsProdOutMin=[]  UdiffTsProdOutMax=[]  NTsProdOutMin=[]  NTsProdOutMax=[]  UintegralTsProdOutMin=[]  UintegralTsProdOutMax=[]  UngainTsProdOutMin=[]  UngainTsProdOutMax=[]  ClampingZeroOutDataTypeStr=Inherit: Inherit via back propagation  ClampingZeroOutMin=[]  ClampingZeroOutMax=[]  FilterDenConstantOutDataTypeStr=Inherit: Inherit via back propagation  FilterDenConstantOutMin=[]  FilterDenConstantOutMax=[]  PCopyOutDataTypeStr=Inherit: Inherit via back propagation  PCopyOutMin=[]  PCopyOutMax=[]  NCopyOutDataTypeStr=Inherit: Inherit via back propagation  NCopyOutMin=[]  NCopyOutMax=[]  IntegratorContinuousStateAttributes=''  IntegratorStateMustResolveToSignalObject=off  IntegratorRTWStateStorageClass=Auto  FilterContinuousStateAttributes=''  FilterStateMustResolveToSignalObject=off  FilterRTWStateStorageClass=Auto  ParallelPVariant=InternalParameters  IdealPVariant=Disabled  IVariant=InternalParameters  DVariant=InternalParameters  IntegratorVariant=Discrete  SatVariant=Disabled  AWVariant=Passthrough  PCopyVariant=Disabled  TRVariant=Disabled  FdbkBlocksVariant=Forward  IdealPFdbkVariant=Disabled  SatFdbkVariant=Disabled  DerivativeFilterVariant=ForwardEulerFilter  NVariant=InternalParameters  NCopyVariant=Disabled  FilterICVariant=InternalICsFilter  IntegratorICVariant=InternalICs  ExternalResetVariant=Disabled  TRSumVariant=Passthrough  SumFdbkVariant=Disabled  SumVariant=Sum_PID  TsampFilterVariant=InternalTs  TsampNgainVariant=Passthrough  TsampIntegralVariant=Passthrough  ExternalSaturationOutDataTypeStr=Inherit: Same as second input
  Output2 : Outport
  wires:
  Discrete Transfer Fcn/1 -> Output2/1
  PID Controller/1 -> Discrete Transfer Fcn/1
  u/1 -> PID Controller/1

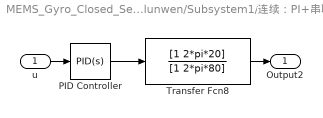
== system MEMS_Gyro_Closed_SenseMode_yangchenglunwen/Subsystem1/连续：PI+串联校正器2 ==
  u : Inport
  PID Controller : slpidlib/PID Controller  Controller=PID  Form=Parallel  TimeDomain=Continuous-time  UseExternalTs=off  SampleTime=-1  IntegratorMethod=Forward Euler  FilterMethod=Forward Euler  ControllerParametersSource=internal  P=0.9  I=2*pi*18  UseKiTs=off  D=0  N=100  UseFilter=on  TunerSelectOption=Transfer Function Based (PID Tuner App)  InitialConditionSource=internal  InitialConditionForIntegrator=0  InitialConditionForFilter=0  DifferentiatorICPrevScaledInput=0  ExternalReset=none  TrackingMode=off  Kt=1  LimitOutput=off  SatLimitsSource=internal  UpperSaturationLimit=inf  LowerSaturationLimit=-inf  LinearizeAsGain=on  AntiWindupMode=none  Kb=1  LimitIntegrator=off  UpperIntegratorSaturationLimit=inf  LowerIntegratorSaturationLimit=-inf  POutMin=[]  POutMax=[]  IOutMin=[]  IOutMax=[]  DOutMin=[]  DOutMax=[]  NOutMin=[]  NOutMax=[]  SumOutMin=[]  SumOutMax=[]  SaturationOutMin=[]  SaturationOutMax=[]  PParamMin=[]  PParamMax=[]  IParamMin=[]  IParamMax=[]  DParamMin=[]  DParamMax=[]  NParamMin=[]  NParamMax=[]  KbParamMin=[]  KbParamMax=[]  KtParamMin=[]  KtParamMax=[]  KbOutMin=[]  KbOutMax=[]  KtOutMin=[]  KtOutMax=[]  IntegratorOutMin=[]  IntegratorOutMax=[]  FilterOutMin=[]  FilterOutMax=[]  SumI1OutMin=[]  SumI1OutMax=[]  SumI2OutMin=[]  SumI2OutMax=[]  SumI3OutMin=[]  SumI3OutMax=[]  SumI4OutMin=[]  SumI4OutMax=[]  SumDOutMin=[]  SumDOutMax=[]  DifferentiatorOutMin=[]  DifferentiatorOutMax=[]  FilterDiffOutCoefMin=[]  FilterDiffOutCoefMax=[]  ReciprocalOutMin=[]  ReciprocalOutMax=[]  SumDenOutMin=[]  SumDenOutMax=[]  SumNumOutMin=[]  SumNumOutMax=[]  DivideOutMin=[]  DivideOutMax=[]  UdiffTsProdOutMin=[]  UdiffTsProdOutMax=[]  NTsProdOutMin=[]  NTsProdOutMax=[]  UintegralTsProdOutMin=[]  UintegralTsProdOutMax=[]  UngainTsProdOutMin=[]  UngainTsProdOutMax=[]  ClampingZeroOutDataTypeStr=Inherit: Inherit via back propagation  ClampingZeroOutMin=[]  ClampingZeroOutMax=[]  FilterDenConstantOutDataTypeStr=Inherit: Inherit via back propagation  FilterDenConstantOutMin=[]  FilterDenConstantOutMax=[]  PCopyOutDataTypeStr=Inherit: Inherit via back propagation  PCopyOutMin=[]  PCopyOutMax=[]  NCopyOutDataTypeStr=Inherit: Inherit via back propagation  NCopyOutMin=[]  NCopyOutMax=[]  IntegratorContinuousStateAttributes=''  IntegratorStateMustResolveToSignalObject=off  IntegratorRTWStateStorageClass=Auto  FilterContinuousStateAttributes=''  FilterStateMustResolveToSignalObject=off  FilterRTWStateStorageClass=Auto  ParallelPVariant=InternalParameters  IdealPVariant=Disabled  IVariant=InternalParameters  DVariant=InternalParameters  IntegratorVariant=Continuous  SatVariant=Disabled  AWVariant=Passthrough  PCopyVariant=Disabled  TRVariant=Disabled  FdbkBlocksVariant=Forward  IdealPFdbkVariant=Disabled  SatFdbkVariant=Disabled  DerivativeFilterVariant=ContFilter  NVariant=InternalParameters  NCopyVariant=Disabled  FilterICVariant=InternalICsFilter  IntegratorICVariant=InternalICs  ExternalResetVariant=Disabled  TRSumVariant=Passthrough  SumFdbkVariant=Disabled  SumVariant=Sum_PID  TsampFilterVariant=InternalTs  TsampNgainVariant=Passthrough  TsampIntegralVariant=Passthrough  ExternalSaturationOutDataTypeStr=Inherit: Same as second input
  Transfer Fcn8 : TransferFcn  Numerator=[1 2*pi*20]  Denominator=[1 2*pi*80]
  Output2 : Outport
  wires:
  u/1 -> PID Controller/1
  PID Controller/1 -> Transfer Fcn8/1
  Transfer Fcn8/1 -> Output2/1

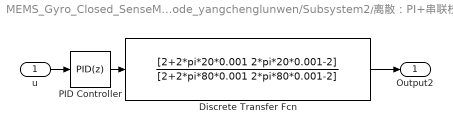
== system MEMS_Gyro_Closed_SenseMode_yangchenglunwen/Subsystem2/离散：PI+串联校正器2 ==
  u : Inport
  Discrete Transfer Fcn : DiscreteTransferFcn  Numerator=[2+2*pi*20*0.001 2*pi*20*0.001-2]  Denominator=[2+2*pi*80*0.001 2*pi*80*0.001-2]  SampleTime=1/1000
  PID Controller : slpidlib/PID Controller  Controller=PID  Form=Parallel  TimeDomain=Discrete-time  UseExternalTs=off  SampleTime=1/1000  IntegratorMethod=Forward Euler  FilterMethod=Forward Euler  ControllerParametersSource=internal  P=0.9  I=2*pi*18  UseKiTs=off  D=0  N=100  UseFilter=on  TunerSelectOption=Transfer Function Based (PID Tuner App)  InitialConditionSource=internal  InitialConditionForIntegrator=0  InitialConditionForFilter=0  DifferentiatorICPrevScaledInput=0  ExternalReset=none  TrackingMode=off  Kt=1  LimitOutput=off  SatLimitsSource=internal  UpperSaturationLimit=inf  LowerSaturationLimit=-inf  LinearizeAsGain=on  AntiWindupMode=none  Kb=1  LimitIntegrator=off  UpperIntegratorSaturationLimit=inf  LowerIntegratorSaturationLimit=-inf  POutMin=[]  POutMax=[]  IOutMin=[]  IOutMax=[]  DOutMin=[]  DOutMax=[]  NOutMin=[]  NOutMax=[]  SumOutMin=[]  SumOutMax=[]  SaturationOutMin=[]  SaturationOutMax=[]  PParamMin=[]  PParamMax=[]  IParamMin=[]  IParamMax=[]  DParamMin=[]  DParamMax=[]  NParamMin=[]  NParamMax=[]  KbParamMin=[]  KbParamMax=[]  KtParamMin=[]  KtParamMax=[]  KbOutMin=[]  KbOutMax=[]  KtOutMin=[]  KtOutMax=[]  IntegratorOutMin=[]  IntegratorOutMax=[]  FilterOutMin=[]  FilterOutMax=[]  SumI1OutMin=[]  SumI1OutMax=[]  SumI2OutMin=[]  SumI2OutMax=[]  SumI3OutMin=[]  SumI3OutMax=[]  SumI4OutMin=[]  SumI4OutMax=[]  SumDOutMin=[]  SumDOutMax=[]  DifferentiatorOutMin=[]  DifferentiatorOutMax=[]  FilterDiffOutCoefMin=[]  FilterDiffOutCoefMax=[]  ReciprocalOutMin=[]  ReciprocalOutMax=[]  SumDenOutMin=[]  SumDenOutMax=[]  SumNumOutMin=[]  SumNumOutMax=[]  DivideOutMin=[]  DivideOutMax=[]  UdiffTsProdOutMin=[]  UdiffTsProdOutMax=[]  NTsProdOutMin=[]  NTsProdOutMax=[]  UintegralTsProdOutMin=[]  UintegralTsProdOutMax=[]  UngainTsProdOutMin=[]  UngainTsProdOutMax=[]  ClampingZeroOutDataTypeStr=Inherit: Inherit via back propagation  ClampingZeroOutMin=[]  ClampingZeroOutMax=[]  FilterDenConstantOutDataTypeStr=Inherit: Inherit via back propagation  FilterDenConstantOutMin=[]  FilterDenConstantOutMax=[]  PCopyOutDataTypeStr=Inherit: Inherit via back propagation  PCopyOutMin=[]  PCopyOutMax=[]  NCopyOutDataTypeStr=Inherit: Inherit via back propagation  NCopyOutMin=[]  NCopyOutMax=[]  IntegratorContinuousStateAttributes=''  IntegratorStateMustResolveToSignalObject=off  IntegratorRTWStateStorageClass=Auto  FilterContinuousStateAttributes=''  FilterStateMustResolveToSignalObject=off  FilterRTWStateStorageClass=Auto  ParallelPVariant=InternalParameters  IdealPVariant=Disabled  IVariant=InternalParameters  DVariant=InternalParameters  IntegratorVariant=Discrete  SatVariant=Disabled  AWVariant=Passthrough  PCopyVariant=Disabled  TRVariant=Disabled  FdbkBlocksVariant=Forward  IdealPFdbkVariant=Disabled  SatFdbkVariant=Disabled  DerivativeFilterVariant=ForwardEulerFilter  NVariant=InternalParameters  NCopyVariant=Disabled  FilterICVariant=InternalICsFilter  IntegratorICVariant=InternalICs  ExternalResetVariant=Disabled  TRSumVariant=Passthrough  SumFdbkVariant=Disabled  SumVariant=Sum_PID  TsampFilterVariant=InternalTs  TsampNgainVariant=Passthrough  TsampIntegralVariant=Passthrough  ExternalSaturationOutDataTypeStr=Inherit: Same as second input
  Output2 : Outport
  wires:
  Discrete Transfer Fcn/1 -> Output2/1
  PID Controller/1 -> Discrete Transfer Fcn/1
  u/1 -> PID Controller/1

== system MEMS_Gyro_Closed_SenseMode_yangchenglunwen/Subsystem2/连续：PI+串联校正器2 ==
  u : Inport
  PID Controller : slpidlib/PID Controller  Controller=PID  Form=Parallel  TimeDomain=Continuous-time  UseExternalTs=off  SampleTime=-1  IntegratorMethod=Forward Euler  FilterMethod=Forward Euler  ControllerParametersSource=internal  P=0.9  I=2*pi*18  UseKiTs=off  D=0  N=100  UseFilter=on  TunerSelectOption=Transfer Function Based (PID Tuner App)  InitialConditionSource=internal  InitialConditionForIntegrator=0  InitialConditionForFilter=0  DifferentiatorICPrevScaledInput=0  ExternalReset=none  TrackingMode=off  Kt=1  LimitOutput=off  SatLimitsSource=internal  UpperSaturationLimit=inf  LowerSaturationLimit=-inf  LinearizeAsGain=on  AntiWindupMode=none  Kb=1  LimitIntegrator=off  UpperIntegratorSaturationLimit=inf  LowerIntegratorSaturationLimit=-inf  POutMin=[]  POutMax=[]  IOutMin=[]  IOutMax=[]  DOutMin=[]  DOutMax=[]  NOutMin=[]  NOutMax=[]  SumOutMin=[]  SumOutMax=[]  SaturationOutMin=[]  SaturationOutMax=[]  PParamMin=[]  PParamMax=[]  IParamMin=[]  IParamMax=[]  DParamMin=[]  DParamMax=[]  NParamMin=[]  NParamMax=[]  KbParamMin=[]  KbParamMax=[]  KtParamMin=[]  KtParamMax=[]  KbOutMin=[]  KbOutMax=[]  KtOutMin=[]  KtOutMax=[]  IntegratorOutMin=[]  IntegratorOutMax=[]  FilterOutMin=[]  FilterOutMax=[]  SumI1OutMin=[]  SumI1OutMax=[]  SumI2OutMin=[]  SumI2OutMax=[]  SumI3OutMin=[]  SumI3OutMax=[]  SumI4OutMin=[]  SumI4OutMax=[]  SumDOutMin=[]  SumDOutMax=[]  DifferentiatorOutMin=[]  DifferentiatorOutMax=[]  FilterDiffOutCoefMin=[]  FilterDiffOutCoefMax=[]  ReciprocalOutMin=[]  ReciprocalOutMax=[]  SumDenOutMin=[]  SumDenOutMax=[]  SumNumOutMin=[]  SumNumOutMax=[]  DivideOutMin=[]  DivideOutMax=[]  UdiffTsProdOutMin=[]  UdiffTsProdOutMax=[]  NTsProdOutMin=[]  NTsProdOutMax=[]  UintegralTsProdOutMin=[]  UintegralTsProdOutMax=[]  UngainTsProdOutMin=[]  UngainTsProdOutMax=[]  ClampingZeroOutDataTypeStr=Inherit: Inherit via back propagation  ClampingZeroOutMin=[]  ClampingZeroOutMax=[]  FilterDenConstantOutDataTypeStr=Inherit: Inherit via back propagation  FilterDenConstantOutMin=[]  FilterDenConstantOutMax=[]  PCopyOutDataTypeStr=Inherit: Inherit via back propagation  PCopyOutMin=[]  PCopyOutMax=[]  NCopyOutDataTypeStr=Inherit: Inherit via back propagation  NCopyOutMin=[]  NCopyOutMax=[]  IntegratorContinuousStateAttributes=''  IntegratorStateMustResolveToSignalObject=off  IntegratorRTWStateStorageClass=Auto  FilterContinuousStateAttributes=''  FilterStateMustResolveToSignalObject=off  FilterRTWStateStorageClass=Auto  ParallelPVariant=InternalParameters  IdealPVariant=Disabled  IVariant=InternalParameters  DVariant=InternalParameters  IntegratorVariant=Continuous  SatVariant=Disabled  AWVariant=Passthrough  PCopyVariant=Disabled  TRVariant=Disabled  FdbkBlocksVariant=Forward  IdealPFdbkVariant=Disabled  SatFdbkVariant=Disabled  DerivativeFilterVariant=ContFilter  NVariant=InternalParameters  NCopyVariant=Disabled  FilterICVariant=InternalICsFilter  IntegratorICVariant=InternalICs  ExternalResetVariant=Disabled  TRSumVariant=Passthrough  SumFdbkVariant=Disabled  SumVariant=Sum_PID  TsampFilterVariant=InternalTs  TsampNgainVariant=Passthrough  TsampIntegralVariant=Passthrough  ExternalSaturationOutDataTypeStr=Inherit: Same as second input
  Transfer Fcn8 : TransferFcn  Numerator=[1 2*pi*20]  Denominator=[1 2*pi*80]
  Output2 : Outport
  wires:
  u/1 -> PID Controller/1
  PID Controller/1 -> Transfer Fcn8/1
  Transfer Fcn8/1 -> Output2/1

== matlab function MEMS_Gyro_Closed_SenseMode_yangchenglunwen/MATLAB Function2 ==
  data: u input; y output
function y = fcn(u)
% w=10*2*pi*(u-2);
% if(u<2)
%     y= 100/360*2*pi;
% else
%     y = 100/360*2*pi*cos(w*(u-2));
%     %y = 100/360*2*pi*cos(2*pi*10*(u-2));
% end
w=0.5*2*pi;
y = 100/360*2*pi*cos(w*u);
